simulink model "lab1ex7"  (Simulink 6.0)
settings: Solver=ode45  StartTime=0.0  StopTime=10.0  RelTol=1e-3
settings Model: LastModifiedBy=student

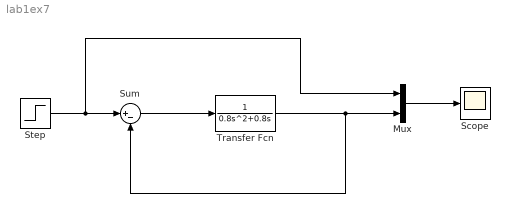
== system lab1ex7 ==
  Mux : Mux  Inputs=2
  Scope : Scope
  Step : Step  SampleTime=0
  Sum : Sum  Inputs=|+-
  Transfer Fcn : TransferFcn  Denominator=[0.8 0.8 0]
  wires:
  Step/1 -> Sum/1, Mux/1
  Sum/1 -> Transfer Fcn/1
  Transfer Fcn/1 -> Mux/2, Sum/2
  Mux/1 -> Scope/1
